simulink model "fuzzy_model"  (R2022b)
settings: Solver=FixedStepAuto  StartTime=0.0  StopTime=t_end  FixedStep=0.1  RelTol=1e-3
undefined symbols (not defined in the file): d_time, d_val, delay, den, Kd, Ki, Kp, Ku, num, r_time, r_val, sel, Ts, u_max, u_min
libraries: fuzblock x2
settings Model: Creator=Milosh Yokich  LastModifiedBy=Milosh Yokich
settings DataIOCC: ReturnWorkspaceOutputs=off

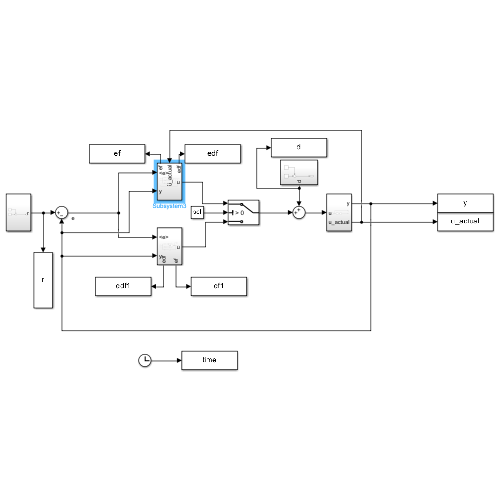
[thumbnail: Simulink's stored preview of the top-level diagram]
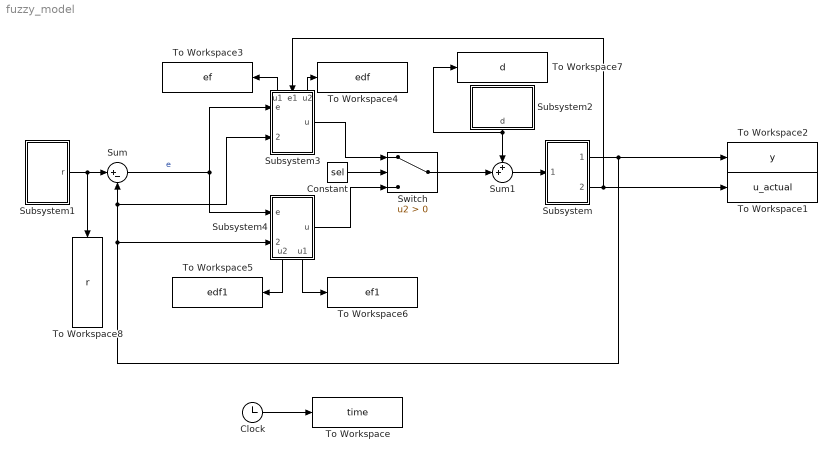
== system fuzzy_model ==
  Clock : Clock
  Constant : Constant  Value=sel
  Subsystem : Subsystem
  Subsystem1 : Subsystem
  Subsystem2 : Subsystem
  Subsystem3 : Subsystem
      settings: PortSchema="{\"entries\":[{\"content\":{\"sides\":[{\"content\":{\"connectorIds\":[\"In1\",\"In2\"]},\"type\":\"ConnectorPlacement.EquallySpacedRectSide\",\"uuid\":\"54f93994-89b5-48d6-a7fd-e34b162a6dcd\"},{\"content\":{\"connectorIds\":[\"Out1\"],\"side\":\"RIGHT\"},\"type\":\"ConnectorPlacement.EquallySpacedRectSide\",\"uuid\":\"2b02b8d4-bf78-4526-b00b-81f8b64abe06\"},{\"content\":{\"connectorIds\":[\"Out2\",\"In3\",\"Out3\"],\"side\":\"TOP\"},\"type\":\"ConnectorPlacement.EquallySpacedRectSide\",\"uuid\":\"2634f88c-e8ee-4590-ad5d-937a6f0bf3f3\"}]},\"type\":\"ConnectorPlacement.EquallySpacedConnector\",\"uuid\":\"917b2687-79c7-43f4-84ad-6326b1ac21bc\"}],\"packageUris\":[\"http://schema.mathworks.com/mf0/Connector/R2020b\"],\"version\":\"1.0\"}"
  Subsystem4 : Subsystem
      settings: PortSchema="{\"entries\":[{\"content\":{\"sides\":[{\"content\":{\"connectorIds\":[\"In1\",\"In2\"]},\"type\":\"ConnectorPlacement.EquallySpacedRectSide\",\"uuid\":\"54f93994-89b5-48d6-a7fd-e34b162a6dcd\"},{\"content\":{\"connectorIds\":[\"Out1\"],\"side\":\"RIGHT\"},\"type\":\"ConnectorPlacement.EquallySpacedRectSide\",\"uuid\":\"2b02b8d4-bf78-4526-b00b-81f8b64abe06\"},{\"content\":{\"connectorIds\":[],\"side\":\"TOP\"},\"type\":\"ConnectorPlacement.EquallySpacedRectSide\",\"uuid\":\"2634f88c-e8ee-4590-ad5d-937a6f0bf3f3\"},{\"content\":{\"connectorIds\":[\"Out2\",\"Out3\"],\"side\":\"BOTTOM\"},\"type\":\"ConnectorPlacement.EquallySpacedRectSide\",\"uuid\":\"93e32108-6ba4-469c-8e7e-ce5dd18f0586\"}]},\"type\":\"ConnectorPlacement.EquallySpacedConnector\",\"uuid\":\"917b2687-79c7-43f4-84ad-6326b1ac21bc\"}],\"packageUris\":[\"http://schema.mathworks.com/mf0/Connector/R2020b\"],\"version\":\"1.0\"}"
  Sum : Sum  Inputs=|+-
  Sum1 : Sum  Inputs=++|
  Switch : Switch  Criteria=u2 > Threshold  SaturateOnIntegerOverflow=off  InputSameDT=off
  To Workspace : ToWorkspace  VariableName=time  SampleTime=-1
  To Workspace1 : ToWorkspace  VariableName=u_actual  SampleTime=-1
  To Workspace2 : ToWorkspace  VariableName=y  SampleTime=-1
  To Workspace3 : ToWorkspace  VariableName=ef  SampleTime=-1
  To Workspace4 : ToWorkspace  VariableName=edf  SampleTime=-1
  To Workspace5 : ToWorkspace  VariableName=edf1  SampleTime=-1
  To Workspace6 : ToWorkspace  VariableName=ef1  SampleTime=-1
  To Workspace7 : ToWorkspace  VariableName=d  SampleTime=-1
  To Workspace8 : ToWorkspace  VariableName=r  SampleTime=-1
  wires:
  Subsystem1/1(r) -> To Workspace8/1, Sum/1
  Subsystem/1(Out1) -> To Workspace2/1, Subsystem4/2(Input), Subsystem3/2(Input), Sum/2
  Subsystem2/1(d) -> Sum1/1, To Workspace7/1
  Sum1/1 -> Subsystem/1(In1)
  Clock/1 -> To Workspace/1
  Subsystem/2(Out2) -> Subsystem3/3(e1), To Workspace1/1
  Subsystem3/2(u1) -> To Workspace3/1
  Subsystem3/3(u2) -> To Workspace4/1
  Subsystem4/3(u1) -> To Workspace6/1
  Subsystem4/2(u2) -> To Workspace5/1
  Sum/1 -> Subsystem4/1(e), Subsystem3/1(e)  "e"
  Subsystem3/1(u) -> Switch/1
  Switch/1 -> Sum1/2
  Constant/1 -> Switch/2
  Subsystem4/1(u) -> Switch/3

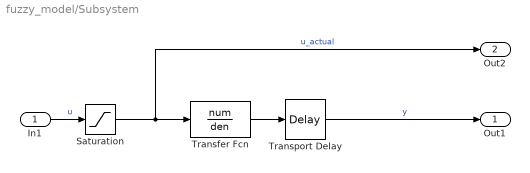
== system fuzzy_model/Subsystem ==
  In1 : Inport
  Saturation : Saturate  UpperLimit=u_max  LowerLimit=u_min
  Transfer Fcn : TransferFcn  Numerator=num  Denominator=den
  Transport Delay : TransportDelay  DelayTime=Ts
  Out1 : Outport
  Out2 : Outport  Port=2
  wires:
  In1/1 -> Saturation/1  "u"
  Transfer Fcn/1 -> Transport Delay/1
  Transport Delay/1 -> Out1/1  "y"
  Saturation/1 -> Out2/1, Transfer Fcn/1  "u_actual"

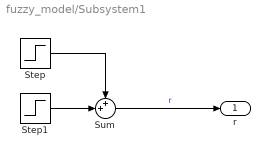
== system fuzzy_model/Subsystem1 ==
  Step : Step  Time=r_time  After=-r_val  SampleTime=0
  Step1 : Step  Time=r_time+delay  After=r_val*2  SampleTime=0
  Sum : Sum  Inputs=++|
  r : Outport
  wires:
  Step/1 -> Sum/1
  Step1/1 -> Sum/2
  Sum/1 -> r/1  "r"

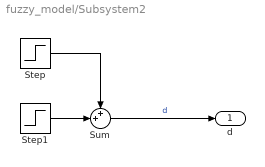
== system fuzzy_model/Subsystem2 ==
  Step : Step  Time=d_time  After=d_val  SampleTime=0
  Step1 : Step  Time=d_time+delay  After=-2*d_val  SampleTime=0
  Sum : Sum  Inputs=++|
  d : Outport
  wires:
  Step/1 -> Sum/1
  Step1/1 -> Sum/2
  Sum/1 -> d/1  "d"

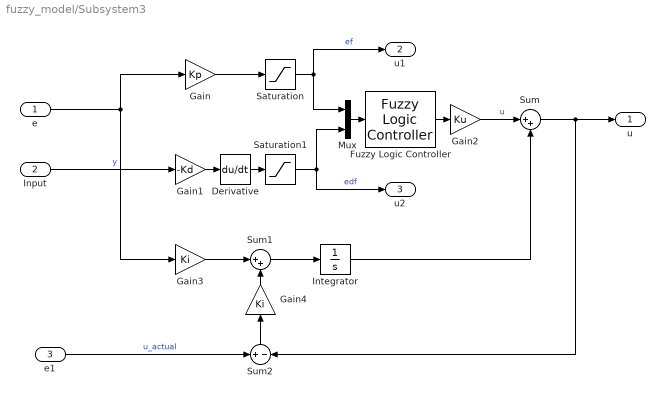
== system fuzzy_model/Subsystem3 ==
  e : Inport
  Input : Inport  Port=2
  e1 : Inport  Port=3
  Derivative : Derivative  CoefficientInTFapproximation=Tf
  Fuzzy Logic Controller : fuzblock/Fuzzy Logic  Controller  FIS='rules.fis'  OutputSampleNumber=101  DataType=double  FuzzifiedInputs=off  RuleFiringStrengths=off  RuleOutputs=off  AggregatedOutputs=off  SimulateUsing=Code generation  OutOfRangeInputValueMessage=none  NoRuleFiredMessage=none  EmptyOutputFuzzySetMessage=none
  Gain : Gain  Gain=Kp
  Gain1 : Gain  Gain=-Kd
  Gain2 : Gain  Gain=Ku
  Gain3 : Gain  Gain=Ki
  Gain4 : Gain  Gain=Ki
  Integrator : Integrator
  Mux : Mux  Inputs=2
  Saturation : Saturate  UpperLimit=1  LowerLimit=-1
  Saturation1 : Saturate  UpperLimit=1  LowerLimit=-1
  Sum : Sum  Inputs=|++
  Sum1 : Sum  Inputs=|++
  Sum2 : Sum  Inputs=+|-
  u : Outport
  u1 : Outport  Port=2
  u2 : Outport  Port=3
  wires:
  Mux/1 -> Fuzzy Logic Controller/1
  e/1 -> Gain3/1, Gain/1
  Saturation/1 -> u1/1, Mux/1  "ef"
  Fuzzy Logic Controller/1 -> Gain2/1
  Saturation1/1 -> Mux/2, u2/1  "edf"
  Derivative/1 -> Saturation1/1
  Gain/1 -> Saturation/1
  Gain1/1 -> Derivative/1
  Gain2/1 -> Sum/1  "u"
  Sum/1 -> Sum2/2, u/1
  Integrator/1 -> Sum/2
  Gain3/1 -> Sum1/1
  Sum1/1 -> Integrator/1
  Gain4/1 -> Sum1/2
  Sum2/1 -> Gain4/1
  e1/1 -> Sum2/1  "u_actual"
  Input/1 -> Gain1/1  "y"

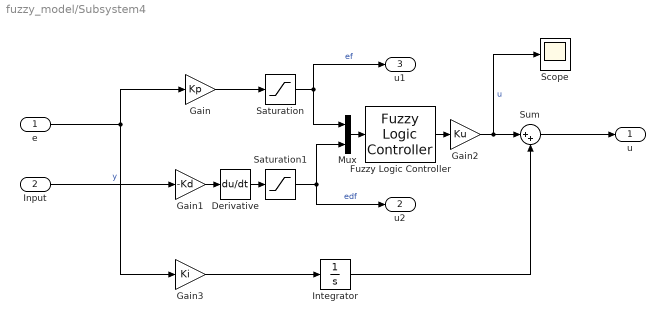
== system fuzzy_model/Subsystem4 ==
  e : Inport
  Input : Inport  Port=2
  Derivative : Derivative  CoefficientInTFapproximation=Tf
  Fuzzy Logic Controller : fuzblock/Fuzzy Logic  Controller  FIS='rules.fis'  OutputSampleNumber=101  DataType=double  FuzzifiedInputs=off  RuleFiringStrengths=off  RuleOutputs=off  AggregatedOutputs=off  SimulateUsing=Code generation  OutOfRangeInputValueMessage=none  NoRuleFiredMessage=none  EmptyOutputFuzzySetMessage=none
  Gain : Gain  Gain=Kp
  Gain1 : Gain  Gain=-Kd
  Gain2 : Gain  Gain=Ku
  Gain3 : Gain  Gain=Ki
  Integrator : Integrator
  Mux : Mux  Inputs=2
  Saturation : Saturate  UpperLimit=1  LowerLimit=-1
  Saturation1 : Saturate  UpperLimit=1  LowerLimit=-1
  Scope : Scope
  Sum : Sum  Inputs=|++
  u : Outport
  u2 : Outport  Port=2
  u1 : Outport  Port=3
  wires:
  Mux/1 -> Fuzzy Logic Controller/1
  e/1 -> Gain3/1, Gain/1
  Saturation/1 -> u1/1, Mux/1  "ef"
  Fuzzy Logic Controller/1 -> Gain2/1
  Saturation1/1 -> Mux/2, u2/1  "edf"
  Derivative/1 -> Saturation1/1
  Gain/1 -> Saturation/1
  Gain1/1 -> Derivative/1
  Gain2/1 -> Scope/1, Sum/1  "u"
  Sum/1 -> u/1
  Integrator/1 -> Sum/2
  Gain3/1 -> Integrator/1
  Input/1 -> Gain1/1  "y"
